simulink library "DC_GRIDSIM_LIB_v1"  (R2022b)
settings: Solver=VariableStepAuto  StartTime=0.0  StopTime=10.0  RelTol=1e-3
undefined symbols (not defined in the file or in its folder): Allday_timevector, High, Household1_Autumnallday, Household1_Springallday, Household1_Summerallday, Household1_Winterallday, Low, MV
libraries: fl_lib x22, nesl_utility x20, simulink x4, ee_lib x3
settings Model: Creator=cfn2169  LastModifiedBy=mingreico

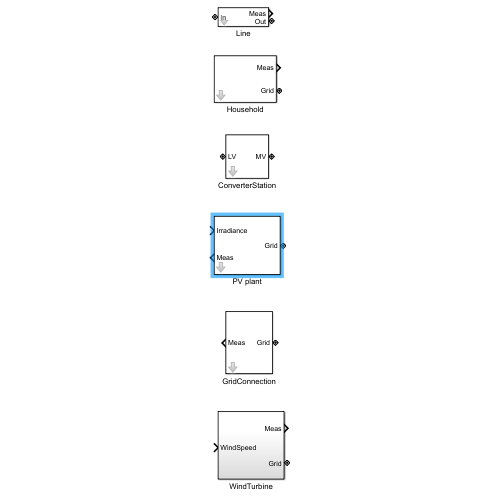
[thumbnail: Simulink's stored preview of the top-level diagram]
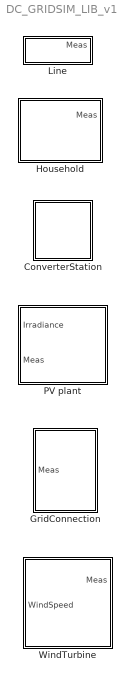
== system DC_GRIDSIM_LIB_v1 ==
  ConverterStation : Subsystem  mask{LV_Ref=380}
      mask prompts: LV_Ref "Nominal voltage of LV side"
      mask DialogControl DescTextVar Prompt: Model of a MVDC/LVDC converter station
  GridConnection : Subsystem  mask{MV_Ref=10000}
      mask prompts: MV_Ref "MV voltage reference"
  Household : Subsystem  mask{ProfileSpring=Household1_Springallday, ProfileSummer=Household1_Summerallday, ProfileAutumn=Household1_Autumnallday, ProfileWinter=Household1_Winterallday, Timevector=Allday_timevector, k=1, VnomLoad=380}
      mask prompts: ProfileSpring "Load profile for spring"; ProfileSummer "Load profile for summer"; ProfileAutumn "Load profile for autumn"; ProfileWinter "Load profile for winter"; Timevector "Corresponding timevector"; k "Scaling factor"; VnomLoad "Nominal voltage load"
      mask DialogControl DescTextVar Prompt: Profile-based load model for households
  Line : Subsystem  mask{rho=1.68e-8, l=1.0, A=240e-6}
      mask prompts: rho "Specific resistivity in Ohm*m"; l "Length in m"; A "Cross sectional area in m^2"
      mask DialogControl DescTextVar Prompt: Resistive line model for two-wired DC systems
  PV plant : Subsystem  mask{eta_pv=0.2, area_pv=1000}
      mask prompts: eta_pv "Efficiency of PV modules"; area_pv "Effective area of PV modules in m^2"
      settings: PortSchema="{\"entries\":[{\"content\":{\"sides\":[{\"content\":{\"connectorIds\":[\"LConn1\"]},\"type\":\"ConnectorPlacement.EquallySpacedRectSide\",\"uuid\":\"e7d30e91-d877-4849-85d5-5068117b5a73\"},{\"content\":{\"connectorIds\":[\"In1\",\"Out1\"],\"side\":\"RIGHT\"},\"type\":\"ConnectorPlacement.EquallySpacedRectSide\",\"uuid\":\"aff2ec47-1e97-401e-aec0-02d86814fbc3\"},{\"content\":{\"connectorIds\":[],\"side\":\"TOP\"},\"type\":\"ConnectorPlacement.EquallySpacedRectSide\",\"uuid\":\"0abfbb66-97f7-400f-9c84-fe1e10d1a17f\"}]},\"type\":\"ConnectorPlacement.EquallySpacedConnector\",\"uuid\":\"740b86aa-7ace-499a-bee9-62f02e790000\"}],\"packageUris\":[\"http://schema.mathworks.com/mf0/Connector/R2020b\"],\"version\":\"1.0\"}"
  WindTurbine : Subsystem

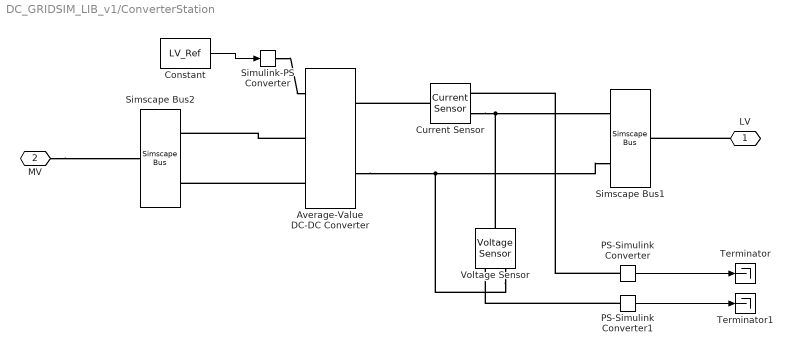
== system DC_GRIDSIM_LIB_v1/ConverterStation ==
  Average-Value DC-DC Converter : ee_lib/Semiconductors & Converters/Converters/Average-Value DC-DC Converter  control_option=ee.enum.converters.controlinput.voltage  converter_type=ee.enum.converters.dcdctype.buck  efficiency_option=ee.enum.converters.efficiency.constant  efficiency_fixed=100  i_vec=[0, 2, 5] A  efficiency_vec=[90, 95, 98]
      settings: InternalSimscapePortConfiguration="{\"Bottom\":[],\"Left\":[{\"id\":\"Vref\",\"label\":\"Vref\",\"type\":\"input\"},{\"id\":\"p1\",\"label\":\"1+\",\"type\":\"foundation.electrical.electrical\"},{\"id\":\"n1\",\"label\":\"1-\",\"type\":\"foundation.electrical.electrical\"}],\"Right\":[{\"id\":\"p2\",\"label\":\"2+\",\"type\":\"foundation.electrical.electrical\"},{\"id\":\"n2\",\"label\":\"2-\",\"type\":\"foundation.electrical.electrical\"}],\"Top\":[]}"
  Constant : Constant  Value=LV_Ref
  Current Sensor : fl_lib/Electrical/Electrical Sensors/Current Sensor
  PS-Simulink Converter : nesl_utility/PS-Simulink Converter  PhysicalDomain=network_engine_domain  SubClassName=ps_output  LeftPortType=input  RightPortType=output  PseudoPeriodic=off  Frequencies=[]  VectorFormat=inherit  Unit=inherit  AffineConversion=off
  PS-Simulink Converter1 : nesl_utility/PS-Simulink Converter  PhysicalDomain=network_engine_domain  SubClassName=ps_output  LeftPortType=input  RightPortType=output  PseudoPeriodic=off  Frequencies=[]  VectorFormat=inherit  Unit=inherit  AffineConversion=off
  Simscape Bus1 : SimscapeBus  HierarchyStrings=High;Low
  Simscape Bus2 : SimscapeBus  HierarchyStrings=High;Low
  Simulink-PS Converter : nesl_utility/Simulink-PS Converter  PhysicalDomain=network_engine_domain  SubClassName=ps_input  LeftPortType=input  RightPortType=output  PseudoPeriodic=off  Frequencies=[]  NoiseDistribution=none  NoiseParameters=[]  Unit=1  AffineConversion=off  FilteringAndDerivatives=provide  SimscapeFilterOrder=1  InputFilterTimeConstant=0.001  UdotUserProvided=0
  Terminator : Terminator
  Terminator1 : Terminator
  Voltage Sensor : fl_lib/Electrical/Electrical Sensors/Voltage Sensor
  LV : PMIOPort  Side=Left
  MV : PMIOPort  Port=2  Side=Right
  wires:
  PS-Simulink Converter/1 -> Terminator/1
  PS-Simulink Converter1/1 -> Terminator1/1
  Constant/1 -> Simulink-PS Converter/1
  connections:
  Voltage Sensor/RConn2 -- Simscape Bus1/LConn2 -- Average-Value DC-DC Converter/RConn2
  Voltage Sensor/LConn1 -- Simscape Bus1/LConn1 -- Current Sensor/RConn2
  Current Sensor/LConn1 -- Average-Value DC-DC Converter/RConn1
  PS-Simulink Converter/LConn1 -- Current Sensor/RConn1
  Average-Value DC-DC Converter/LConn2 -- Simscape Bus2/LConn1
  Average-Value DC-DC Converter/LConn3 -- Simscape Bus2/LConn2
  Simulink-PS Converter/RConn1 -- Average-Value DC-DC Converter/LConn1
  PS-Simulink Converter1/LConn1 -- Voltage Sensor/RConn1
  LV/RConn1 -- Simscape Bus1/RConn1
  MV/RConn1 -- Simscape Bus2/RConn1

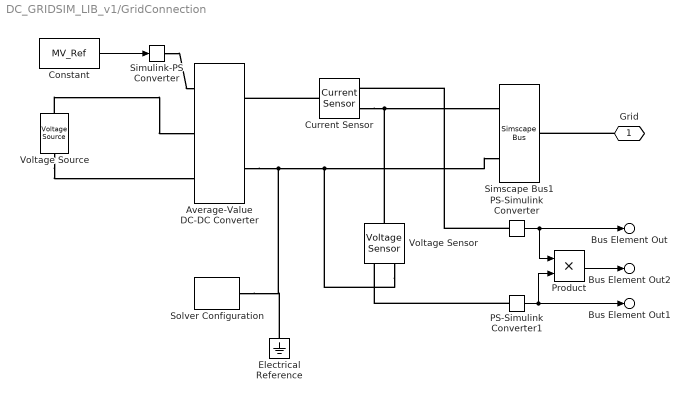
== system DC_GRIDSIM_LIB_v1/GridConnection ==
  Average-Value DC-DC Converter : ee_lib/Semiconductors & Converters/Converters/Average-Value DC-DC Converter  control_option=ee.enum.converters.controlinput.voltage  converter_type=ee.enum.converters.dcdctype.buck  efficiency_option=ee.enum.converters.efficiency.constant  efficiency_fixed=100  i_vec=[0, 2, 5] A  efficiency_vec=[90, 95, 98]
      settings: InternalSimscapePortConfiguration="{\"Bottom\":[],\"Left\":[{\"id\":\"Vref\",\"label\":\"Vref\",\"type\":\"input\"},{\"id\":\"p1\",\"label\":\"1+\",\"type\":\"foundation.electrical.electrical\"},{\"id\":\"n1\",\"label\":\"1-\",\"type\":\"foundation.electrical.electrical\"}],\"Right\":[{\"id\":\"p2\",\"label\":\"2+\",\"type\":\"foundation.electrical.electrical\"},{\"id\":\"n2\",\"label\":\"2-\",\"type\":\"foundation.electrical.electrical\"}],\"Top\":[]}"
  Constant : Constant  Value=MV_Ref
  Current Sensor : fl_lib/Electrical/Electrical Sensors/Current Sensor
  Electrical Reference : fl_lib/Electrical/Electrical Elements/Electrical Reference
  PS-Simulink Converter : nesl_utility/PS-Simulink Converter  PhysicalDomain=network_engine_domain  SubClassName=ps_output  LeftPortType=input  RightPortType=output  PseudoPeriodic=off  Frequencies=[]  VectorFormat=inherit  Unit=inherit  AffineConversion=off
  PS-Simulink Converter1 : nesl_utility/PS-Simulink Converter  PhysicalDomain=network_engine_domain  SubClassName=ps_output  LeftPortType=input  RightPortType=output  PseudoPeriodic=off  Frequencies=[]  VectorFormat=inherit  Unit=inherit  AffineConversion=off
  Product : Product
  Simscape Bus1 : SimscapeBus  HierarchyStrings=High;Low
  Simulink-PS Converter : nesl_utility/Simulink-PS Converter  PhysicalDomain=network_engine_domain  SubClassName=ps_input  LeftPortType=input  RightPortType=output  PseudoPeriodic=off  Frequencies=[]  NoiseDistribution=none  NoiseParameters=[]  Unit=1  AffineConversion=off  FilteringAndDerivatives=provide  SimscapeFilterOrder=1  InputFilterTimeConstant=0.001  UdotUserProvided=0
  Solver Configuration : nesl_utility/Solver Configuration  PhysicalDomain=network_engine_domain  SubClassName=solver  LeftPortType=input  RightPortType=generic  Tones=[]  Harmonics=[]  SimulateNoise=off  Profile=off  UseLocalSampling=off  EnableSwitchedLinearOptims=on  FrequencyDomain=off  UseCCode=off  RelTol=0.001  AbsTol=0.001  MinStep=1e-09  ToWorkspace=off  RevertToSquareIcSolve=off  NumHomotopyIterations=100  PhasorMode=off  PhasorModeNumHarmonics=1  ConsistencySolver=NEWTON_XTOL_AFTER_FTOL  IndexReductionMethod=DerivativeReplacement  DoDC=off  ResidualTolerance=1e-09  ConsistencyTolSource=GLOBAL  ConsistencyAbsTol=0.001  ConsistencyRelTol=0.001  ConsistencyTolFactor=0.001  UseLocalSolver=off  LocalSolverChoice=NE_BACKWARD_EULER_ADVANCER  ResolveIndetEquations=on  FunctionEvalNumThread=1  LocalSolverSampleTime=0.001  DoFixedCost=off  MaxNonlinIter=3  MaxModeIter=2  ComputeImpulses=off  ImpulseIterations=2  LinearAlgebra=auto  LinearAlgebraNumThread=0  EquationFormulation=NE_TIME_EF  DelaysMemoryBudget=1024  AutomaticFiltering=on  FilteringTimeConstant=0.001  PartitionStorageMethod=AS_NEEDED  PartitionMemoryBudget=1024  PartitionMethod=ROBUST
  Voltage Sensor : fl_lib/Electrical/Electrical Sensors/Voltage Sensor
  Voltage Source : ee_lib/Sources/Voltage Source  dc_voltage=10000 V  ac_voltage=0 V  ac_shift=0 rad  ac_frequency=60 Hz  noise_mode=ee.enum.sources.noise.Disabled  PSD=0 V^2/Hz  sample_time=1e-3 s  repeatability=ee.enum.sources.repeatability.NotRepeatable  user_seed=0  auto_seed=3499211588  i_specify=off  i_priority=None  i=0 A  i_nominal_specify=off  i_nominal_unit=A  i_nominal_value=1  v_specify=off  v_priority=None  v=0 V  v_nominal_specify=off  v_nominal_unit=V  v_nominal_value=1
  Grid : PMIOPort  Side=Left
  Bus Element Out : Outport  PortName=Meas  Element=Current
  Bus Element Out1 : Outport  PortName=Meas  Element=Voltage
  Bus Element Out2 : Outport  PortName=Meas  Element=Power
  wires:
  Constant/1 -> Simulink-PS Converter/1
  PS-Simulink Converter/1 -> Product/1, Bus Element Out/1
  PS-Simulink Converter1/1 -> Product/2, Bus Element Out1/1
  Product/1 -> Bus Element Out2/1
  connections:
  Grid/RConn1 -- Simscape Bus1/RConn1
  Voltage Source/LConn1 -- Average-Value DC-DC Converter/LConn2
  Voltage Source/RConn1 -- Average-Value DC-DC Converter/LConn3
  Simulink-PS Converter/RConn1 -- Average-Value DC-DC Converter/LConn1
  Average-Value DC-DC Converter/RConn2 -- Solver Configuration/RConn1 -- Electrical Reference/LConn1 -- Voltage Sensor/RConn2 -- Simscape Bus1/LConn2
  Current Sensor/RConn2 -- Voltage Sensor/LConn1 -- Simscape Bus1/LConn1
  Current Sensor/LConn1 -- Average-Value DC-DC Converter/RConn1
  PS-Simulink Converter1/LConn1 -- Voltage Sensor/RConn1
  PS-Simulink Converter/LConn1 -- Current Sensor/RConn1

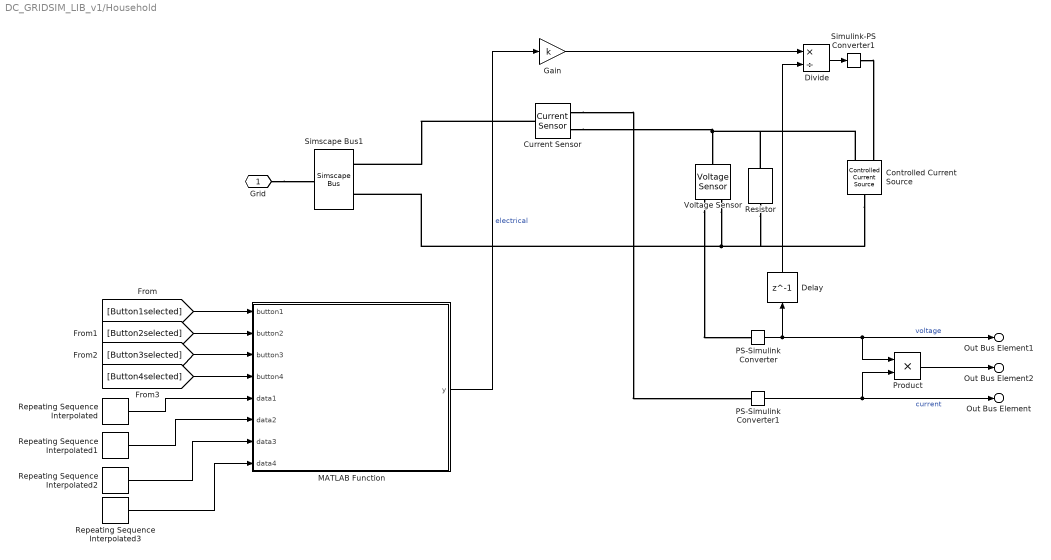
== system DC_GRIDSIM_LIB_v1/Household ==
  Controlled Current Source : fl_lib/Electrical/Electrical Sources/Controlled Current Source
  Current Sensor : fl_lib/Electrical/Electrical Sensors/Current Sensor
  Delay : Delay  DelayLength=1  InitialCondition=VnomLoad
  Divide : Product  Inputs=*/
  Gain : Gain  Gain=k
  MATLAB Function : MATLAB Function  TreatAsAtomicUnit=on
  PS-Simulink Converter : nesl_utility/PS-Simulink Converter  PhysicalDomain=network_engine_domain  SubClassName=ps_output  LeftPortType=input  RightPortType=output  PseudoPeriodic=off  Frequencies=[]  VectorFormat=inherit  Unit=inherit  AffineConversion=off
  PS-Simulink Converter1 : nesl_utility/PS-Simulink Converter  PhysicalDomain=network_engine_domain  SubClassName=ps_output  LeftPortType=input  RightPortType=output  PseudoPeriodic=off  Frequencies=[]  VectorFormat=inherit  Unit=inherit  AffineConversion=off
  Product : Product
  Repeating Sequence Interpolated : simulink/Sources/Repeating Sequence Interpolated  OutValues=ProfileSpring  TimeValues=Timevector  LookUpMeth=Interpolation-Use End Values  tsamp=0.01  OutMin=[]  OutMax=[]  OutDataTypeStr=double  OutputDataTypeScalingMode=double  OutDataType=fixdt(0,8)  OutScaling=2^-10
  Repeating Sequence Interpolated1 : simulink/Sources/Repeating Sequence Interpolated  OutValues=ProfileSummer  TimeValues=Timevector  LookUpMeth=Interpolation-Use End Values  tsamp=0.01  OutMin=[]  OutMax=[]  OutDataTypeStr=double  OutputDataTypeScalingMode=double  OutDataType=fixdt(0,8)  OutScaling=2^-10
  Repeating Sequence Interpolated2 : simulink/Sources/Repeating Sequence Interpolated  OutValues=ProfileAutumn  TimeValues=Timevector  LookUpMeth=Interpolation-Use End Values  tsamp=0.01  OutMin=[]  OutMax=[]  OutDataTypeStr=double  OutputDataTypeScalingMode=double  OutDataType=fixdt(0,8)  OutScaling=2^-10
  Repeating Sequence Interpolated3 : simulink/Sources/Repeating Sequence Interpolated  OutValues=ProfileWinter  TimeValues=Timevector  LookUpMeth=Interpolation-Use End Values  tsamp=0.01  OutMin=[]  OutMax=[]  OutDataTypeStr=double  OutputDataTypeScalingMode=double  OutDataType=fixdt(0,8)  OutScaling=2^-10
  Resistor : fl_lib/Electrical/Electrical Elements/Resistor  R=1e9 Ohm  i_specify=off  i_priority=None  i=0 A  i_nominal_specify=off  i_nominal_unit=A  i_nominal_value=1  v_specify=off  v_priority=None  v=0 V  v_nominal_specify=off  v_nominal_unit=V  v_nominal_value=1
  Simscape Bus1 : SimscapeBus  HierarchyStrings=High;Low
  Simulink-PS Converter1 : nesl_utility/Simulink-PS Converter  PhysicalDomain=network_engine_domain  SubClassName=ps_input  LeftPortType=input  RightPortType=output  PseudoPeriodic=off  Frequencies=[]  NoiseDistribution=none  NoiseParameters=[]  Unit=A  AffineConversion=off  FilteringAndDerivatives=provide  SimscapeFilterOrder=1  InputFilterTimeConstant=0.001  UdotUserProvided=0
  Voltage Sensor : fl_lib/Electrical/Electrical Sensors/Voltage Sensor
  Grid : PMIOPort  Side=Right
  Out Bus Element : Outport  PortName=Meas  Element=Current
  Out Bus Element1 : Outport  PortName=Meas  Element=Voltage
  Out Bus Element2 : Outport  PortName=Meas  Element=Power
  wires:
  MATLAB Function/1(y) -> Gain/1  "electrical"
  PS-Simulink Converter/1 -> Product/1, Out Bus Element1/1, Delay/1  "voltage"
  PS-Simulink Converter1/1 -> Product/2, Out Bus Element/1  "current"
  [Button4selected] -> MATLAB Function/4(button4)
  [Button3selected] -> MATLAB Function/3(button3)
  [Button2selected] -> MATLAB Function/2(button2)
  [Button1selected] -> MATLAB Function/1(button1)
  Repeating Sequence Interpolated/1 -> MATLAB Function/5(data1)
  Repeating Sequence Interpolated1/1 -> MATLAB Function/6(data2)
  Repeating Sequence Interpolated2/1 -> MATLAB Function/7(data3)
  Repeating Sequence Interpolated3/1 -> MATLAB Function/8(data4)
  Product/1 -> Out Bus Element2/1
  Gain/1 -> Divide/1
  Divide/1 -> Simulink-PS Converter1/1
  Delay/1 -> Divide/2
  connections:
  Grid/RConn1 -- Simscape Bus1/RConn1
  Voltage Sensor/RConn2 -- Resistor/RConn1 -- Controlled Current Source/LConn1 -- Simscape Bus1/LConn2
  Voltage Sensor/RConn1 -- PS-Simulink Converter/LConn1
  Current Sensor/RConn1 -- PS-Simulink Converter1/LConn1
  Current Sensor/LConn1 -- Simscape Bus1/LConn1
  Current Sensor/RConn2 -- Resistor/LConn1 -- Controlled Current Source/RConn2 -- Voltage Sensor/LConn1
  Simulink-PS Converter1/RConn1 -- Controlled Current Source/RConn1

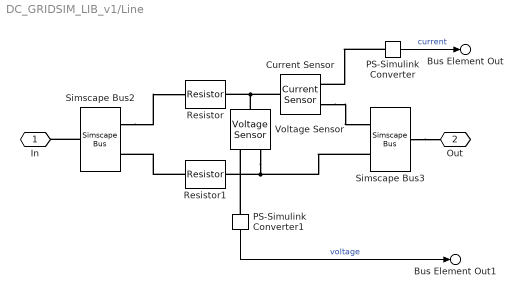
== system DC_GRIDSIM_LIB_v1/Line ==
  Current Sensor : fl_lib/Electrical/Electrical Sensors/Current Sensor
  PS-Simulink Converter : nesl_utility/PS-Simulink Converter  PhysicalDomain=network_engine_domain  SubClassName=ps_output  LeftPortType=input  RightPortType=output  PseudoPeriodic=off  Frequencies=[]  VectorFormat=inherit  Unit=inherit  AffineConversion=off
  PS-Simulink Converter1 : nesl_utility/PS-Simulink Converter  PhysicalDomain=network_engine_domain  SubClassName=ps_output  LeftPortType=input  RightPortType=output  PseudoPeriodic=off  Frequencies=[]  VectorFormat=inherit  Unit=inherit  AffineConversion=off
  Resistor : fl_lib/Electrical/Electrical Elements/Resistor  R=rho*l/A Ohm  i_specify=off  i_priority=None  i=0 A  i_nominal_specify=off  i_nominal_unit=A  i_nominal_value=1  v_specify=off  v_priority=None  v=0 V  v_nominal_specify=off  v_nominal_unit=V  v_nominal_value=1
  Resistor1 : fl_lib/Electrical/Electrical Elements/Resistor  R=rho*l/A Ohm  i_specify=off  i_priority=None  i=0 A  i_nominal_specify=off  i_nominal_unit=A  i_nominal_value=1  v_specify=off  v_priority=None  v=0 V  v_nominal_specify=off  v_nominal_unit=V  v_nominal_value=1
  Simscape Bus2 : SimscapeBus  HierarchyStrings=High;Low
  Simscape Bus3 : SimscapeBus  HierarchyStrings=High;Low
  Voltage Sensor : fl_lib/Electrical/Electrical Sensors/Voltage Sensor
  In : PMIOPort  Side=Left
  Out : PMIOPort  Port=2  Side=Right
  Bus Element Out : Outport  PortName=Meas  Element=current
  Bus Element Out1 : Outport  PortName=Meas  Element=voltage
  wires:
  PS-Simulink Converter/1 -> Bus Element Out/1  "current"
  PS-Simulink Converter1/1 -> Bus Element Out1/1  "voltage"
  connections:
  Simscape Bus2/LConn1 -- Resistor/LConn1
  Simscape Bus3/LConn2 -- Voltage Sensor/RConn2 -- Resistor1/RConn1
  Simscape Bus2/RConn1 -- In/RConn1
  Resistor1/LConn1 -- Simscape Bus2/LConn2
  Simscape Bus3/RConn1 -- Out/RConn1
  Current Sensor/LConn1 -- Voltage Sensor/LConn1 -- Resistor/RConn1
  Current Sensor/RConn2 -- Simscape Bus3/LConn1
  PS-Simulink Converter/LConn1 -- Current Sensor/RConn1
  PS-Simulink Converter1/LConn1 -- Voltage Sensor/RConn1

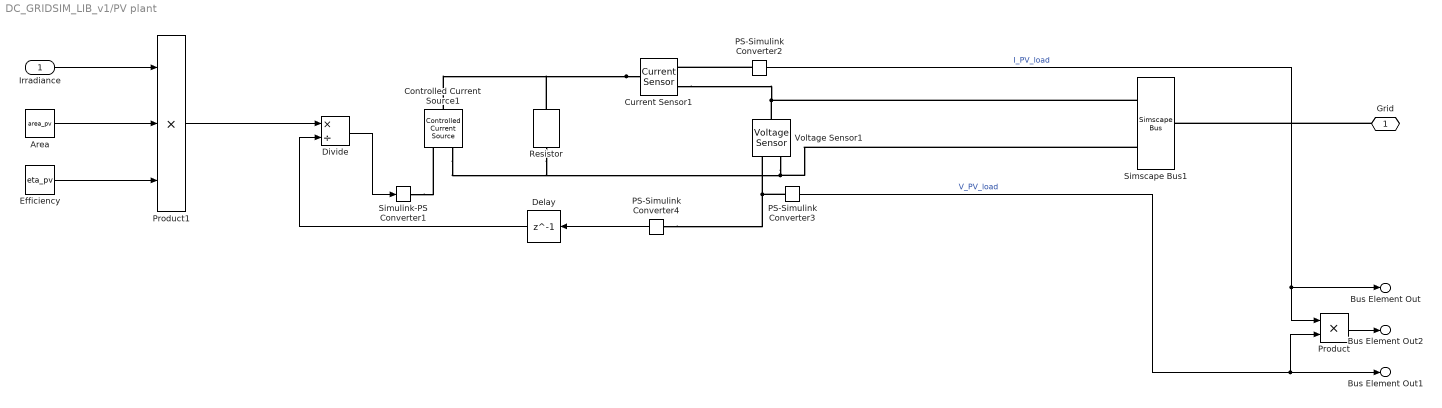
== system DC_GRIDSIM_LIB_v1/PV plant ==
  Irradiance : Inport
  Area : Constant  Value=area_pv
  Controlled Current Source1 : fl_lib/Electrical/Electrical Sources/Controlled Current Source
  Current Sensor1 : fl_lib/Electrical/Electrical Sensors/Current Sensor
  Delay : Delay  DelayLength=1  InitialCondition=MV
  Divide : Product  Inputs=*/
  Efficiency : Constant  Value=eta_pv
  PS-Simulink Converter2 : nesl_utility/PS-Simulink Converter  PhysicalDomain=network_engine_domain  SubClassName=ps_output  LeftPortType=input  RightPortType=output  PseudoPeriodic=off  Frequencies=[]  VectorFormat=1-D array  Unit=inherit  AffineConversion=off
  PS-Simulink Converter3 : nesl_utility/PS-Simulink Converter  PhysicalDomain=network_engine_domain  SubClassName=ps_output  LeftPortType=input  RightPortType=output  PseudoPeriodic=off  Frequencies=[]  VectorFormat=1-D array  Unit=inherit  AffineConversion=off
  PS-Simulink Converter4 : nesl_utility/PS-Simulink Converter  PhysicalDomain=network_engine_domain  SubClassName=ps_output  LeftPortType=input  RightPortType=output  PseudoPeriodic=off  Frequencies=[]  VectorFormat=inherit  Unit=inherit  AffineConversion=off
  Product : Product
  Product1 : Product  Inputs=3
  Resistor : fl_lib/Electrical/Electrical Elements/Resistor  R=1e9 Ohm  i_specify=off  i_priority=None  i=0 A  i_nominal_specify=off  i_nominal_unit=A  i_nominal_value=1  v_specify=off  v_priority=None  v=0 V  v_nominal_specify=off  v_nominal_unit=V  v_nominal_value=1
  Simscape Bus1 : SimscapeBus  HierarchyStrings=High;Low
  Simulink-PS Converter1 : nesl_utility/Simulink-PS Converter  PhysicalDomain=network_engine_domain  SubClassName=ps_input  LeftPortType=input  RightPortType=output  PseudoPeriodic=off  Frequencies=[]  NoiseDistribution=none  NoiseParameters=[]  Unit=A  AffineConversion=off  FilteringAndDerivatives=provide  SimscapeFilterOrder=1  InputFilterTimeConstant=0.001  UdotUserProvided=0
  Voltage Sensor1 : fl_lib/Electrical/Electrical Sensors/Voltage Sensor
  Grid : PMIOPort  Side=Left
  Bus Element Out : Outport  PortName=Meas  Element=Current
  Bus Element Out1 : Outport  PortName=Meas  Element=Voltage
  Bus Element Out2 : Outport  PortName=Meas  Element=Power
  wires:
  Area/1 -> Product1/2
  Efficiency/1 -> Product1/3
  Irradiance/1 -> Product1/1
  Delay/1 -> Divide/2
  Divide/1 -> Simulink-PS Converter1/1
  PS-Simulink Converter3/1 -> Product/2, Bus Element Out1/1  "V_PV_load"
  PS-Simulink Converter4/1 -> Delay/1
  Product1/1 -> Divide/1
  PS-Simulink Converter2/1 -> Product/1, Bus Element Out/1  "I_PV_load"
  Product/1 -> Bus Element Out2/1
  connections:
  Grid/RConn1 -- Simscape Bus1/RConn1
  Current Sensor1/LConn1 -- Controlled Current Source1/LConn1 -- Resistor/LConn1
  Voltage Sensor1/RConn2 -- Simscape Bus1/LConn2 -- Resistor/RConn1 -- Controlled Current Source1/RConn2
  Voltage Sensor1/LConn1 -- Simscape Bus1/LConn1 -- Current Sensor1/RConn2
  PS-Simulink Converter4/LConn1 -- PS-Simulink Converter3/LConn1 -- Voltage Sensor1/RConn1
  Simulink-PS Converter1/RConn1 -- Controlled Current Source1/RConn1
  PS-Simulink Converter2/LConn1 -- Current Sensor1/RConn1

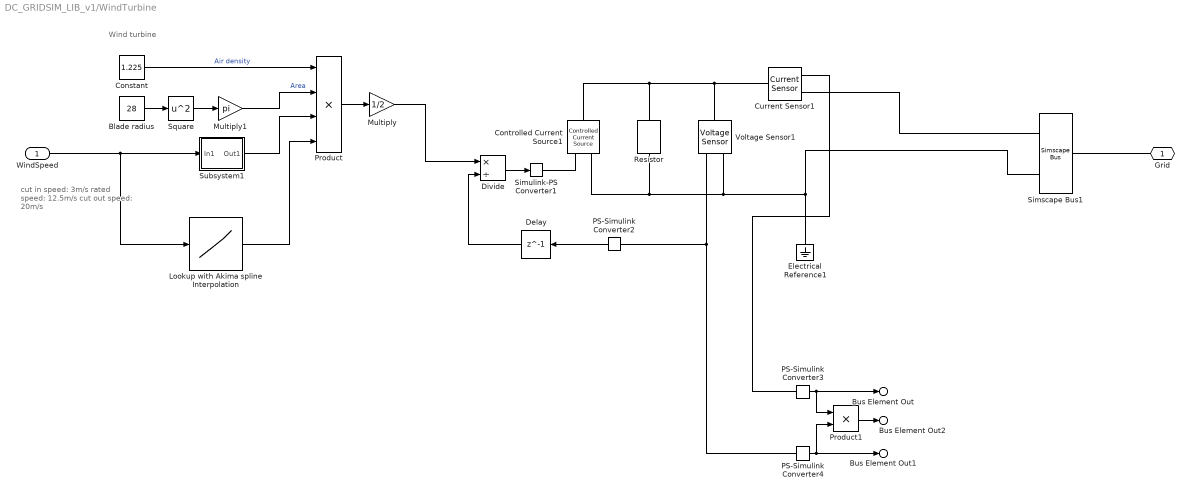
== system DC_GRIDSIM_LIB_v1/WindTurbine ==
  note: cut in speed: 3m/s
      | rated speed: 12.5m/s
      | cut out speed: 20m/s
  note: Wind turbine
  WindSpeed : Inport
  Blade radius : Constant  Value=28
  Constant : Constant  Value=1.225
  Controlled Current Source1 : fl_lib/Electrical/Electrical Sources/Controlled Current Source
  Current Sensor1 : fl_lib/Electrical/Electrical Sensors/Current Sensor
  Delay : Delay  DelayLength=1  InitialCondition=MV
  Divide : Product  Inputs=*/
  Electrical Reference1 : fl_lib/Electrical/Electrical Elements/Electrical Reference
  Lookup with Akima spline Interpolation : Lookup_n-D  NumberOfTableDimensions=1  BreakpointsForDimension1=[0;1;2;3;4;5;6;7;8;9;10;11;12;13;14;15;16;17;18;19;20;21;22;23;24;25;26;27;28]  Table=[0;0;0;0.228;0.322;0.38;0.408;0.413;0.418;0.419;0.419;0.401;0.378;0.305;0.244;0.199;0.164;0.136;0.115;0.098;0.084;0.072;0.063;0.055;0.048;0.042;0;0;0]  InterpMethod=Akima spline  InternalRulePriority=Speed  OutDataTypeStr=double  RndMeth=Simplest
  Multiply : Gain  Gain=1/2
  Multiply1 : Gain  Gain=pi
  PS-Simulink Converter2 : nesl_utility/PS-Simulink Converter  PhysicalDomain=network_engine_domain  SubClassName=ps_output  LeftPortType=input  RightPortType=output  PseudoPeriodic=off  Frequencies=[]  VectorFormat=inherit  Unit=inherit  AffineConversion=off
  PS-Simulink Converter3 : nesl_utility/PS-Simulink Converter  PhysicalDomain=network_engine_domain  SubClassName=ps_output  LeftPortType=input  RightPortType=output  PseudoPeriodic=off  Frequencies=[]  VectorFormat=inherit  Unit=inherit  AffineConversion=off
  PS-Simulink Converter4 : nesl_utility/PS-Simulink Converter  PhysicalDomain=network_engine_domain  SubClassName=ps_output  LeftPortType=input  RightPortType=output  PseudoPeriodic=off  Frequencies=[]  VectorFormat=inherit  Unit=inherit  AffineConversion=off
  Product : Product  Inputs=4
  Product1 : Product
  Resistor : fl_lib/Electrical/Electrical Elements/Resistor  R=1e9 Ohm  i_specify=off  i_priority=None  i=0 A  i_nominal_specify=off  i_nominal_unit=A  i_nominal_value=1  v_specify=off  v_priority=None  v=0 V  v_nominal_specify=off  v_nominal_unit=V  v_nominal_value=1
  Simscape Bus1 : SimscapeBus  HierarchyStrings=High;Low
  Simulink-PS Converter1 : nesl_utility/Simulink-PS Converter  PhysicalDomain=network_engine_domain  SubClassName=ps_input  LeftPortType=input  RightPortType=output  PseudoPeriodic=off  Frequencies=[]  NoiseDistribution=none  NoiseParameters=[]  Unit=1  AffineConversion=off  FilteringAndDerivatives=provide  SimscapeFilterOrder=1  InputFilterTimeConstant=0.001  UdotUserProvided=0
  Square : Math  Operator=square
  Subsystem1 : Subsystem
      mask Display: disp('Vw^3');
  Voltage Sensor1 : fl_lib/Electrical/Electrical Sensors/Voltage Sensor
  Grid : PMIOPort  Side=Right
  Bus Element Out : Outport  PortName=Meas  Element=Current
  Bus Element Out1 : Outport  PortName=Meas  Element=Voltage
  Bus Element Out2 : Outport  PortName=Meas  Element=Power
  wires:
  Multiply1/1 -> Product/2  "Area"
  Blade radius/1 -> Square/1
  Square/1 -> Multiply1/1
  Constant/1 -> Product/1  "Air density"
  WindSpeed/1 -> Lookup with Akima spline Interpolation/1, Subsystem1/1(In1)
  Product/1 -> Multiply/1
  Subsystem1/1(Out1) -> Product/3
  Delay/1 -> Divide/2
  PS-Simulink Converter4/1 -> Product1/2, Bus Element Out1/1
  Divide/1 -> Simulink-PS Converter1/1
  PS-Simulink Converter3/1 -> Product1/1, Bus Element Out/1
  Multiply/1 -> Divide/1
  PS-Simulink Converter2/1 -> Delay/1
  Product1/1 -> Bus Element Out2/1
  Lookup with Akima spline Interpolation/1 -> Product/4
  connections:
  Grid/RConn1 -- Simscape Bus1/RConn1
  Controlled Current Source1/RConn2 -- Voltage Sensor1/RConn2 -- Simscape Bus1/LConn2 -- Electrical Reference1/LConn1 -- Resistor/RConn1
  Resistor/LConn1 -- Current Sensor1/LConn1 -- Voltage Sensor1/LConn1 -- Controlled Current Source1/LConn1
  PS-Simulink Converter4/LConn1 -- Voltage Sensor1/RConn1 -- PS-Simulink Converter2/LConn1
  PS-Simulink Converter3/LConn1 -- Current Sensor1/RConn1
  Simulink-PS Converter1/RConn1 -- Controlled Current Source1/RConn1
  Simscape Bus1/LConn1 -- Current Sensor1/RConn2

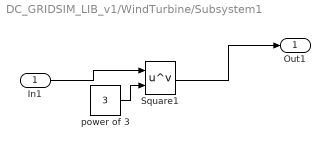
== system DC_GRIDSIM_LIB_v1/WindTurbine/Subsystem1 ==
  In1 : Inport
  Square1 : Math  Operator=pow
  power of 3 : Constant  Value=3
  Out1 : Outport
  wires:
  power of 3/1 -> Square1/2
  Square1/1 -> Out1/1
  In1/1 -> Square1/1

== matlab function DC_GRIDSIM_LIB_v1/Household/MATLAB Function ==
  data: button1 input; button2 input; button3 input; button4 input; data1 input; data2 input; y output; data3 input; data4 input
function y = fcn(button1, button2, button3, button4, data1,data2,data3, data4)
    if button1
        y = data1;
    elseif button2
        y =data2;
    elseif button3
        y = data3;
    elseif button4
        y = data4;
    else 
        y = data1;
    end
end
